simulink model "robot"  (R2016b)
settings: Solver=ode3  StartTime=0.0  StopTime=1000.0  FixedStep=0.2  RelTol=1e-3  EnableMultiTasking=on
undefined symbols (not defined in the file): Angular, Linear
libraries: robotlib x4, simulink x2
settings Model: Creator=esther  LastModifiedBy=esther
settings DataIOCC: SaveFormat=Array
settings OptimizationCC: MaxStackSize=64
settings DebuggingCC: ParameterTunabilityLossMsg=error
settings HardwareCC: ProdBitPerPointer=32  ProdBitPerSizeT=32  ProdBitPerPtrDiffT=32  ProdLargestAtomicFloat=None  ProdIntDivRoundTo=Undefined  ProdEndianess=Unspecified  ProdWordSize=32  ProdHWDeviceType=Generic->Unspecified (assume 32-bit Generic)
settings RTWCC: SystemTargetFile=ert.tlc  HardwareBoard=Robot Operating System (ROS)  TLCOptions="-aInlineSetEventsForThisBaseRateFcn=TLC_FALSE -aSuppressMultiTaskScheduler=TLC_FALSE  -aRateBasedStepFcn=0"  TemplateMakefile=ert_default_tmf  Description=Embedded Coder  GenerateReport=on  Toolchain=Catkin  IncludeHyperlinkInReport=on  LaunchReport=on  TargetLang=C++  GenerateTraceInfo=on  GenerateTraceReport=on  GenerateTraceReportSl=on  GenerateTraceReportSf=on  GenerateTraceReportEml=on
settings CodeAppCC: ForceParamTrailComments=on  OperatorAnnotations=on  SimulinkDataObjDesc=on  SFDataObjDesc=on  MATLABFcnDesc=on  InsertBlockDesc=on  MATLABSourceComments=on
settings ERTTargetCC: MultiInstanceERTCode=on  CodeInterfacePackaging=C++ class  SupportContinuousTime=on  SupportVariableSizeSignals=on  RootIOFormat=Structure reference

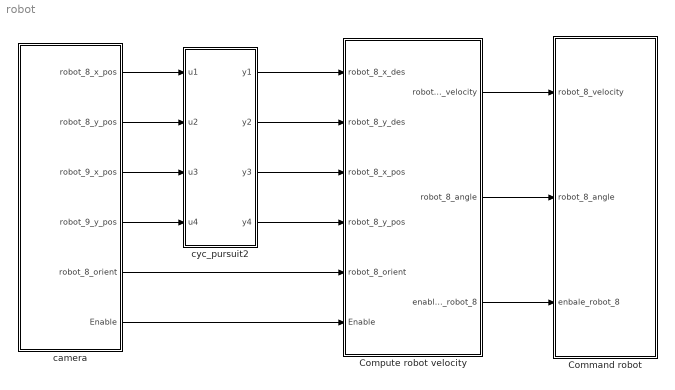
== system robot ==
  Command robot : Subsystem
  Compute robot velocity : Subsystem
  camera : Subsystem
  cyc_pursuit2 : MATLAB Function  TreatAsAtomicUnit=on
  wires:
  camera/1(robot_8_x_pos) -> cyc_pursuit2/1(u1)
  camera/2(robot_8_y_pos) -> cyc_pursuit2/2(u2)
  camera/3(robot_9_x_pos) -> cyc_pursuit2/3(u3)
  camera/4(robot_9_y_pos) -> cyc_pursuit2/4(u4)
  cyc_pursuit2/1(y1) -> Compute robot velocity/1(robot_8_x_des)
  cyc_pursuit2/2(y2) -> Compute robot velocity/2(robot_8_y_des)
  cyc_pursuit2/3(y3) -> Compute robot velocity/3(robot_8_x_pos)
  cyc_pursuit2/4(y4) -> Compute robot velocity/4(robot_8_y_pos)
  camera/5(robot_8_orient) -> Compute robot velocity/5(robot_8_orient)
  camera/6(Enable) -> Compute robot velocity/6(Enable)
  Compute robot velocity/1(robot_8_velocity) -> Command robot/1(robot_8_velocity)
  Compute robot velocity/2(robot_8_angle) -> Command robot/2(robot_8_angle)
  Compute robot velocity/3(enable_robot_8) -> Command robot/3(enbale_robot_8)

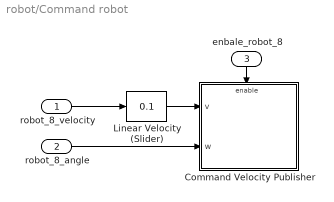
== system robot/Command robot ==
  robot_8_velocity : Inport
  robot_8_angle : Inport  Port=2
  enbale_robot_8 : Inport  Port=3
  Command Velocity Publisher : Subsystem
  Linear Velocity (Slider) : simulink/Math Operations/Slider Gain  low=0  gain=0.1  high=0.2
  wires:
  robot_8_angle/1 -> Command Velocity Publisher/2(w)
  enbale_robot_8/1 -> Command Velocity Publisher/Enable
  robot_8_velocity/1 -> Linear Velocity (Slider)/1
  Linear Velocity (Slider)/1 -> Command Velocity Publisher/1(v)

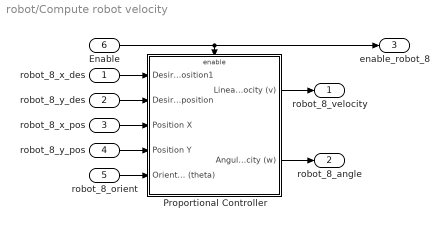
== system robot/Compute robot velocity ==
  robot_8_x_des : Inport
  robot_8_y_des : Inport  Port=2
  robot_8_x_pos : Inport  Port=3
  robot_8_y_pos : Inport  Port=4
  robot_8_orient : Inport  Port=5
  Enable : Inport  Port=6
  Proportional Controller : Subsystem
  robot_8_velocity : Outport
  robot_8_angle : Outport  Port=2
  enable_robot_8 : Outport  Port=3
  wires:
  Proportional Controller/1(Linear Velocity (v)) -> robot_8_velocity/1
  Proportional Controller/2(Angular Velocity (w)) -> robot_8_angle/1
  robot_8_x_pos/1 -> Proportional Controller/3(Position X)
  robot_8_orient/1 -> Proportional Controller/5(Orientation (theta))
  robot_8_x_des/1 -> Proportional Controller/1(Desired position1)
  robot_8_y_pos/1 -> Proportional Controller/4(Position Y)
  robot_8_y_des/1 -> Proportional Controller/2(Desired position)
  Enable/1 -> enable_robot_8/1, Proportional Controller/Enable

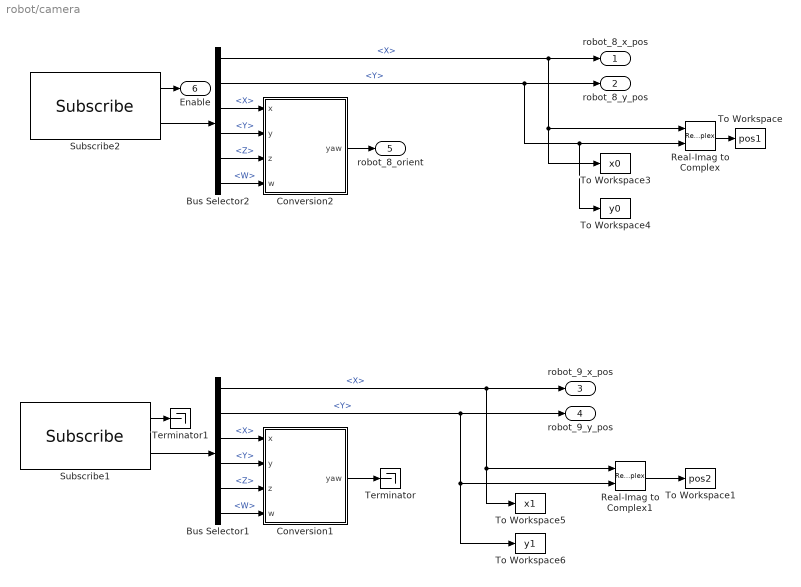
== system robot/camera ==
  Bus Selector1 : BusSelector  OutputSignals=Pose.Position.X,Pose.Position.Y,Pose.Orientation.X,Pose.Orientation.Y,Pose.Orientation.Z,Pose.Orientation.W
  Bus Selector2 : BusSelector  OutputSignals=Pose.Position.X,Pose.Position.Y,Pose.Orientation.X,Pose.Orientation.Y,Pose.Orientation.Z,Pose.Orientation.W
  Conversion1 : MATLAB Function  TreatAsAtomicUnit=on
  Conversion2 : MATLAB Function  TreatAsAtomicUnit=on
  Real-Imag to Complex : RealImagToComplex
  Real-Imag to Complex1 : RealImagToComplex
  Subscribe1 : robotlib/Subscribe  SourceLibraryInfo=This block requires Robotics System Toolbox  topicSource=Select from ROS network  topic=/bot_9/pose  messageType=geometry_msgs/PoseStamped  sampleTime=-1  messageQueueLength=1
  Subscribe2 : robotlib/Subscribe  SourceLibraryInfo=This block requires Robotics System Toolbox  topicSource=Select from ROS network  topic=/bot_8/pose  messageType=geometry_msgs/PoseStamped  sampleTime=-1  messageQueueLength=1
  Terminator : Terminator
  Terminator1 : Terminator
  To Workspace : ToWorkspace  VariableName=pos1  SampleTime=-1
  To Workspace1 : ToWorkspace  VariableName=pos2  SampleTime=-1
  To Workspace3 : ToWorkspace  VariableName=x0  SampleTime=-1
  To Workspace4 : ToWorkspace  VariableName=y0  SampleTime=-1
  To Workspace5 : ToWorkspace  VariableName=x1  SampleTime=-1
  To Workspace6 : ToWorkspace  VariableName=y1  SampleTime=-1
  robot_8_x_pos : Outport
  robot_8_y_pos : Outport  Port=2
  robot_9_x_pos : Outport  Port=3
  robot_9_y_pos : Outport  Port=4
  robot_8_orient : Outport  Port=5
  Enable : Outport  Port=6
  wires:
  Bus Selector2/3 -> Conversion2/1(x)  "<X>"
  Bus Selector2/6 -> Conversion2/4(w)  "<W>"
  Bus Selector2/5 -> Conversion2/3(z)  "<Z>"
  Bus Selector2/4 -> Conversion2/2(y)  "<Y>"
  Subscribe2/2 -> Bus Selector2/1
  Bus Selector1/1 -> Real-Imag to Complex1/1, To Workspace5/1, robot_9_x_pos/1  "<X>"
  Bus Selector1/2 -> Real-Imag to Complex1/2, To Workspace6/1, robot_9_y_pos/1  "<Y>"
  Bus Selector1/3 -> Conversion1/1(x)  "<X>"
  Bus Selector1/4 -> Conversion1/2(y)  "<Y>"
  Bus Selector1/5 -> Conversion1/3(z)  "<Z>"
  Subscribe1/2 -> Bus Selector1/1
  Bus Selector1/6 -> Conversion1/4(w)  "<W>"
  Subscribe2/1 -> Enable/1
  Subscribe1/1 -> Terminator1/1
  Real-Imag to Complex/1 -> To Workspace/1
  Real-Imag to Complex1/1 -> To Workspace1/1
  Conversion1/1(yaw) -> Terminator/1
  Bus Selector2/1 -> robot_8_x_pos/1, Real-Imag to Complex/1, To Workspace3/1  "<X>"
  Bus Selector2/2 -> robot_8_y_pos/1, Real-Imag to Complex/2, To Workspace4/1  "<Y>"
  Conversion2/1(yaw) -> robot_8_orient/1

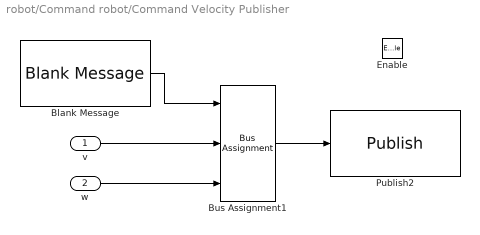
== system robot/Command robot/Command Velocity Publisher ==
  v : Inport
  w : Inport  Port=2
  Enable : EnablePort
  Blank Message : robotlib/Blank Message  SourceLibraryInfo=This block requires Robotics System Toolbox  messageType=geometry_msgs/Twist  SampleTime=inf
  Bus Assignment1 : BusAssignment  DialogController=Simulink.DDGSource_BusAssignment  AssignedSignals=Linear.X,Angular.Z
  Publish2 : robotlib/Publish  SourceLibraryInfo=This block requires Robotics System Toolbox  topicSource=Select from ROS network  topic=/robot_8/cmd_vel  messageType=geometry_msgs/Twist  messageQueueLength=105
  wires:
  Bus Assignment1/1 -> Publish2/1
  Blank Message/1 -> Bus Assignment1/1
  v/1 -> Bus Assignment1/2
  w/1 -> Bus Assignment1/3

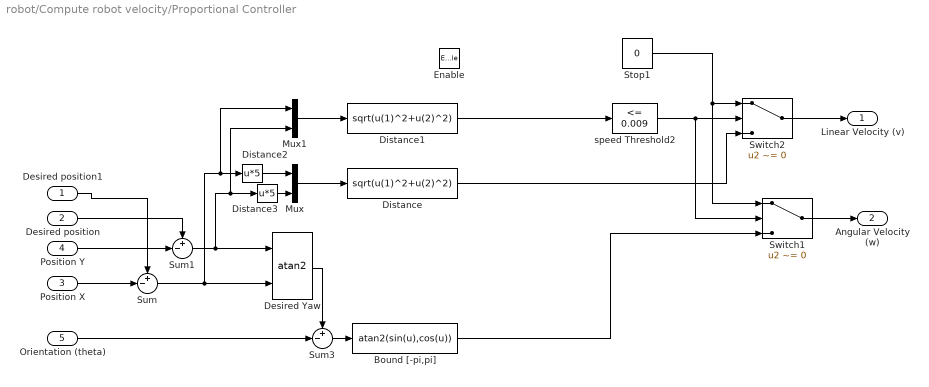
== system robot/Compute robot velocity/Proportional Controller ==
  Desired position1 : Inport
  Desired position : Inport  Port=2
  Position X : Inport  Port=3
  Position Y : Inport  Port=4
  Orientation (theta) : Inport  Port=5
  Enable : EnablePort
  Bound [-pi,pi] : Fcn  Expr=atan2(sin(u),cos(u))
  Desired Yaw : Trigonometry  Operator=atan2
  Distance : Fcn  Expr=sqrt(u(1)^2+u(2)^2)
  Distance1 : Fcn  Expr=sqrt(u(1)^2+u(2)^2)
  Distance2 : Fcn  Expr=u*5
  Distance3 : Fcn  Expr=u*5
  Mux : Mux  Inputs=2
  Mux1 : Mux  Inputs=2
  Stop1 : Constant  Value=0
  Sum : Sum  Inputs=+-|
  Sum1 : Sum  Inputs=+-|
  Sum3 : Sum  Inputs=+-|
  Switch1 : Switch  Criteria=u2 ~= 0
  Switch2 : Switch  Criteria=u2 ~= 0
  speed Threshold2 : simulink/Logic and Bit Operations/Compare To Constant  relop=<=  const=0.009  OutDataTypeStr=boolean
  Linear Velocity (v) : Outport
  Angular Velocity (w) : Outport  Port=2
  wires:
  Desired position1/1 -> Sum/1
  Desired position/1 -> Sum1/1
  Position Y/1 -> Sum1/2
  Position X/1 -> Sum/2
  Mux/1 -> Distance/1
  Orientation (theta)/1 -> Sum3/2
  Desired Yaw/1 -> Sum3/1
  Sum3/1 -> Bound [-pi,pi]/1
  Distance/1 -> Switch2/3
  Distance2/1 -> Mux/1
  Distance3/1 -> Mux/2
  Mux1/1 -> Distance1/1
  Sum/1 -> Desired Yaw/2, Mux1/1, Distance2/1
  Sum1/1 -> Desired Yaw/1, Mux1/2, Distance3/1
  speed Threshold2/1 -> Switch2/2, Switch1/2
  Bound [-pi,pi]/1 -> Switch1/3
  Stop1/1 -> Switch2/1, Switch1/1
  Distance1/1 -> speed Threshold2/1
  Switch1/1 -> Angular Velocity (w)/1
  Switch2/1 -> Linear Velocity (v)/1

== matlab function robot/cyc_pursuit2 ==
  data: u1 input; y1 output; u2 input; u3 input; u4 input; y2 output; y3 output; y4 output
function [y1, y2, y3, y4] = fcn(u1, u2, u3, u4)
%#codegen

y1 = ((1-0.2)*u1+(u3*0.2)+(0.4635*0.2));
y2 = ((1-0.2)*u2+(0.2*u4)-(1.4266*0.2));
y3=u1;
y4=u2;




%       y1 = ((1-0.2)*u1+(u3*0.2)+(1.5451*0.2));
%         y2 = ((1-0.2)*u2+(0.2*u4)+(4.7553*0.2));
%         y3 = ((1-0.2)*u3+(u5*0.2)-(4.0451*0.2));
%         y4 = ((1-0.2)*u4+(u6*0.2)+(2.9389*0.2));
%         y5 = ((1-0.2)*u5+(u7*0.2)-(4.0451*0.2));
%         y6 = ((1-0.2)*u6+(u8*0.2)-(2.9389*0.2));
%         y7 = ((1-0.2)*u7+(u9*0.2)+(1.5451*0.2));
%         y8 = ((1-0.2)*u8+(u10*0.2)-(4.7553*0.2));
%         y9 = ((1-0.2)*u9+(u1*0.2)+(5*0.2));
%         y10 = ((1-0.2)*u10+(u2*0.2)+(0*0.2));

== matlab function robot/camera/Conversion1 ==
  data: yaw output; x input; y input; z input; w input
function yaw  = quat2eul(x,y,z,w)
%#codegen

% Convert the quaternion to a yaw angle (zyx euler angle)
eul = quat2eul([w,x,y,z]);
yaw = eul(1);

end

== matlab function robot/camera/Conversion2 ==
  data: yaw output; x input; y input; z input; w input
function yaw  = quat2eul(x,y,z,w)
%#codegen

% Convert the quaternion to a yaw angle (zyx euler angle)
eul = quat2eul([w,x,y,z]);
yaw = eul(1);

end
